simulink library "unifi_Sil_Lib"  (R2020b)
settings: Solver=VariableStepAuto  StartTime=0.0  StopTime=10.0  RelTol=1e-3
settings Model: Creator=mawal  LastModifiedBy=mawal

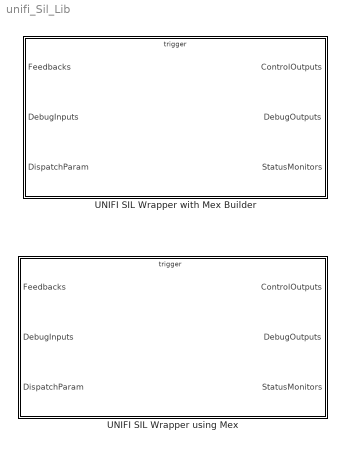
== system unifi_Sil_Lib ==
  UNIFI SIL Wrapper using Mex : Subsystem  TreatAsAtomicUnit=on
      mask DialogControl importSilTemplate Prompt: Step 1: Import SIL template
      mask DialogControl importSilTemplate Callback: cbk_rfMex_import_sil_tem
      mask DialogControl updateInterfaceDim Prompt: Step 2: Update Interface Dimensions
      mask DialogControl updateInterfaceDim Callback: cbk_update_interface_dim
      mask DialogControl buildMexContainer Prompt: Step 3: Setup Mex Container
      mask DialogControl buildMexContainer Callback: cbk_rfMex_setup_mex_container
      mask Display: image('$imagefile'); % Use "Edit Image" on toolstrip to change.
  UNIFI SIL Wrapper with Mex Builder : Subsystem  TreatAsAtomicUnit=on
      mask DialogControl importSilTemplate Prompt: Step 1: Import SIL Template
      mask DialogControl importSilTemplate Callback: cbk_import_sil_tem
      mask DialogControl updateInterfaceDim Prompt: Step 2: Update Interface Dimensions (Add/Link custom code prior to Step 2)
      mask DialogControl updateInterfaceDim Callback: cbk_update_interface_dim
      mask DialogControl configMexBuilder Prompt: Step 3: Configure Mex Builder (Disable Library Link to Enable Self-Modification)
      mask DialogControl configMexBuilder Callback: cbk_setup_mex_builder
      mask DialogControl buildMex Prompt: Step 4: Build Mex
      mask DialogControl buildMex Callback: cbk_build_mex
      mask Display: image('$imagefile'); % Use "Edit Image" on toolstrip to change.

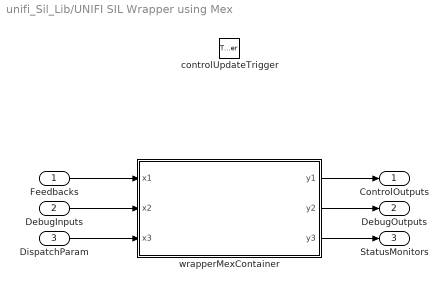
== system unifi_Sil_Lib/UNIFI SIL Wrapper using Mex ==
  Feedbacks : Inport
  DebugInputs : Inport  Port=2
  DispatchParam : Inport  Port=3
  controlUpdateTrigger : TriggerPort  VariantControl=Variant
  wrapperMexContainer : MATLAB Function  TreatAsAtomicUnit=on
  ControlOutputs : Outport
  DebugOutputs : Outport  Port=2
  StatusMonitors : Outport  Port=3
  wires:
  Feedbacks/1 -> wrapperMexContainer/1(x1)
  DebugInputs/1 -> wrapperMexContainer/2(x2)
  DispatchParam/1 -> wrapperMexContainer/3(x3)
  wrapperMexContainer/1(y1) -> ControlOutputs/1
  wrapperMexContainer/2(y2) -> DebugOutputs/1
  wrapperMexContainer/3(y3) -> StatusMonitors/1

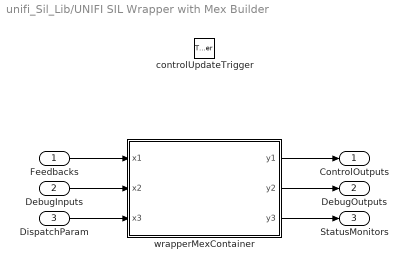
== system unifi_Sil_Lib/UNIFI SIL Wrapper with Mex Builder ==
  Feedbacks : Inport
  DebugInputs : Inport  Port=2
  DispatchParam : Inport  Port=3
  controlUpdateTrigger : TriggerPort  VariantControl=Variant
  wrapperMexContainer : MATLAB Function  TreatAsAtomicUnit=on
  ControlOutputs : Outport
  DebugOutputs : Outport  Port=2
  StatusMonitors : Outport  Port=3
  wires:
  Feedbacks/1 -> wrapperMexContainer/1(x1)
  DebugInputs/1 -> wrapperMexContainer/2(x2)
  DispatchParam/1 -> wrapperMexContainer/3(x3)
  wrapperMexContainer/1(y1) -> ControlOutputs/1
  wrapperMexContainer/2(y2) -> DebugOutputs/1
  wrapperMexContainer/3(y3) -> StatusMonitors/1

== matlab function unifi_Sil_Lib/UNIFI SIL Wrapper using Mex/wrapperMexContainer ==
  data: x1 input; y1 output; x2 input; x3 input; y2 output; y3 output
function [y1, y2, y3] = runWrapperMex(x1, x2, x3)

y1 = x1;
y2 = x2;
y3 = x3;

end

== matlab function unifi_Sil_Lib/UNIFI SIL Wrapper with Mex Builder/wrapperMexContainer ==
  data: x1 input; y1 output; x2 input; x3 input; y2 output; y3 output
function [y1, y2, y3] = runWrapperMex(x1, x2, x3)

y1 = x1;
y2 = x2;
y3 = x3;

end
